simulink model "task1_1"  (R2019b)
settings: Solver=VariableStepAuto  StartTime=0.0  StopTime=10.0  RelTol=1e-3
settings Model: Creator=HUAWEI  LastModifiedBy=HUAWEI

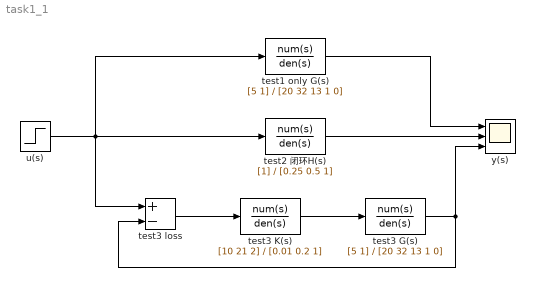
== system task1_1 ==
  test1 only G(s) : TransferFcn  Numerator=[5 1]  Denominator=[20 32 13 1 0]
  test2 闭环H(s) : TransferFcn  Denominator=[0.25 0.5 1]
  test3 G(s) : TransferFcn  Numerator=[5 1]  Denominator=[20 32 13 1 0]
  test3 K(s) : TransferFcn  Numerator=[10 21 2]  Denominator=[0.01 0.2 1]
  test3 loss : Sum  Inputs=+-
  u(s) : Step  SampleTime=0
  y(s) : Scope  NumInputPorts=3
  wires:
  u(s)/1 -> test1 only G(s)/1, test2 闭环H(s)/1, test3 loss/1
  test3 loss/1 -> test3 K(s)/1
  test3 K(s)/1 -> test3 G(s)/1
  test3 G(s)/1 -> y(s)/3, test3 loss/2
  test2 闭环H(s)/1 -> y(s)/2
  test1 only G(s)/1 -> y(s)/1
